simulink model "T37_v65_2015b"  (Simulink 8.6)
settings: Solver=ode45  StartTime=0.0  StopTime=180  FixedStep=0.001  MaxStep=0.1  RelTol=1e-3
values from neighbouring files (symbols this model uses):
  Aero_RP = Aero_RP*[-1 0 0;0 1 0;0 0 -1]    [t37_data.m]
  aileron_limits = [-0.35 0.35]*pi/180    [t37_data.m]
  CD_alpha = 0.3840    (= 0.384)    [t37_data.m]
  CD_beta = [-1.5700	1.2300 ... (first row only)    [t37_data.m]
  CD_flap = 0.0750    (= 0.075)    [t37_data.m]
  CD_zero = [  -1.5700	1.5000 ... (first row only)    [t37_data.m]
  Cl_ail = [0.0000	0.1810 ... (first row only)    [t37_data.m]
  CL_alpha = [-0.2000	-0.6400 ... (first row only)    [t37_data.m]
  CL_alpha_dot = 2.0    (= 2)    [t37_data.m]
  Cl_beta = -0.0944    [t37_data.m]
  CL_elev = 0.5    [t37_data.m]
  CL_flap = 0.3500    (= 0.35)    [t37_data.m]
  CL_ground_effect = [0.0000	1.0610 ... (first row only)    [t37_data.m]
  Cl_p = -0.4420    (= -0.442)    [t37_data.m]
  CL_q = 4.1    [t37_data.m]
  Cl_r = 0.0926    [t37_data.m]
  Cl_rudder = 0.0150    (= 0.015)    [t37_data.m]
  Cm_alpha = -0.7000    (= -0.7)    [t37_data.m]
  Cm_alpha_dot = -6.9500    (= -6.95)    [t37_data.m]
  Cm_elev = [0.0000	-1.1200 ... (first row only)    [t37_data.m]
  Cm_q = -50.0000    (= -50)    [t37_data.m]
  Cm_zero = 0.0250    (= 0.025)    [t37_data.m]
  Cn_beta = 0.1106    [t37_data.m]
  Cn_p = -0.0243    [t37_data.m]
  Cn_r = -0.1390    (= -0.139)    [t37_data.m]
  Cn_rudder = -0.0365    [t37_data.m]
  CY_beta = -0.3460    (= -0.346)    [t37_data.m]
  CY_p = -0.0827    [t37_data.m]
  CY_r = 0.3000    (= 0.3)    [t37_data.m]
  CY_rudder = 0.200    (= 0.2)    [t37_data.m]
  elevator_limits = [-0.35 0.3]*pi/180    [t37_data.m]
  isTrimming = 0    [mytrim.m]    (also in t37_data.m)
  Jxx = 7985*1.3558179    (= 10826.2059315)    [t37_data.m]
  Jxz = 0    [t37_data.m]
  Jyy = 6000*1.3558179    (= 8134.9074)    [t37_data.m]
  Jzz = 11183*1.3558179    (= 15162.1115757)    [t37_data.m]
  M = 4056*0.45359237    (= 1839.77065272)    [t37_data.m]
  Rcg = Rcg*[-1 0 0;0 1 0;0 0 -1]    [t37_data.m]
  Rengine1 = Rengine1*[-1 0 0;0 1 0;0 0 -1]    [t37_data.m]
  Rengine2 = Rengine2*[-1 0 0;0 1 0;0 0 -1]    [t37_data.m]
  rudder_limits = [-0.35 0.35]*pi/180    [t37_data.m]
  Sw = 182*0.09290304    (= 16.90835328)    [t37_data.m]
  thrust_limits = [0 1]    [t37_data.m]
  Tmax = M*10    (= 18397.7065272)    [t37_data.m]
  u0 = [ ... (first row only)    [mytrim.m]    (also in t37_data.m = zeros(4,1))
  x0 = [ ... (first row only)    [mytrim.m]    (also in t37_data.m = zeros(12,1))
undefined symbols (not defined in the file or in its folder): CD_elevator
undefined symbols (not defined in the file): Bw, Cw
(part 1 of 2)
settings Model: Creator=torres  LastModifiedBy=Pc melhor q do euler  ExtModeAutoUpdateStatusClock=off
settings DataIOCC: SaveOutput=off  SaveTime=off  SignalLoggingName=sigsOut
settings OptimizationCC: ExpressionDepthLimit=128  InitFltsAndDblsToZero=on
settings DebuggingCC: SaveWithParameterizedLinksMsg=none  SignalResolutionControl=TryResolveAllWithWarning  SolverPrmCheckMsg=none  MultiTaskDSMMsg=warning  MultiTaskCondExecSysMsg=none  FcnCallInpInsideContextMsg=EnableAllAsWarning  AllowSymbolicDim=on  StateNameClashWarn=none  StrictBusMsg=None
settings HardwareCC: TargetHWDeviceType=32-bit Generic  TargetUnknown=on  ProdEqTarget=off
settings GRTTargetCC: TargetFcnLib=ansi_tfl_tmw.mat  GeneratePreprocessorConditionals=Use local settings

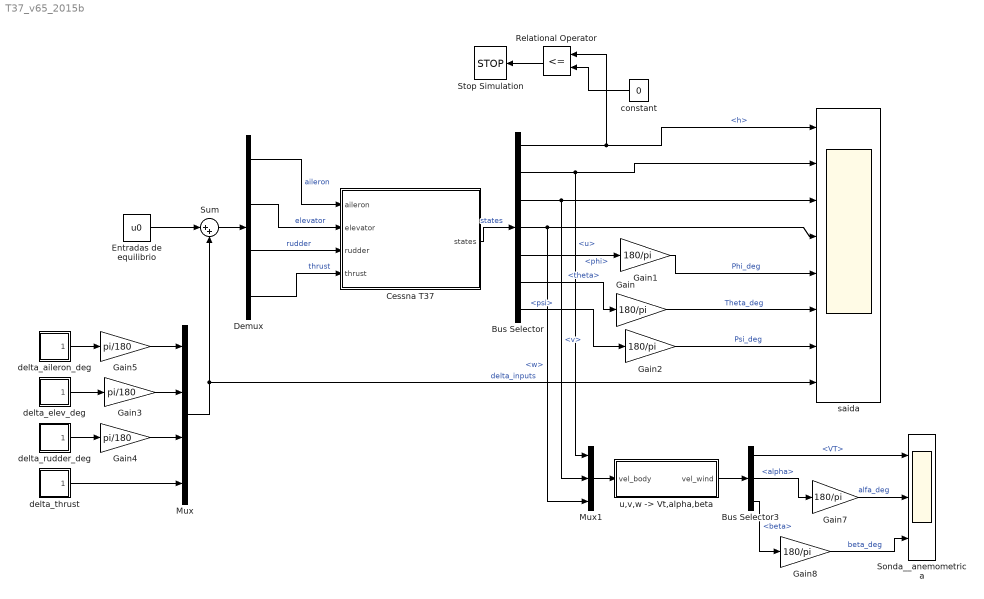
== system T37_v65_2015b ==
  Bus Selector : BusSelector  OutputSignals=h,u,v,w,phi,theta,psi
  Bus Selector3 : BusSelector  OutputSignals=VT,alpha,beta
  Cessna T37 : Subsystem
      mask Display: image(imread('c182.jpg'))
  Demux : Demux
  Entradas de equilibrio : Constant  Value=u0
  Gain{,1..2,7..8} (5 alike) : Gain  Gain=180/pi  SaturateOnIntegerOverflow=on  OutDataTypeStr=Inherit: Same as input  ParamDataTypeStr=Inherit: Same as input
  Gain3 : Gain  Gain=pi/180  SaturateOnIntegerOverflow=on  OutDataTypeStr=Inherit: Same as input  ParamDataTypeStr=Inherit: Same as input
  Gain4 : Gain  Gain=pi/180  SaturateOnIntegerOverflow=on  OutDataTypeStr=Inherit: Same as input  ParamDataTypeStr=Inherit: Same as input
  Gain5 : Gain  Gain=pi/180  SaturateOnIntegerOverflow=on  OutDataTypeStr=Inherit: Same as input  ParamDataTypeStr=Inherit: Same as input
  Mux : Mux
  Mux1 : Mux  Inputs=3
  Relational Operator : RelationalOperator  Operator=<=
  Sonda__anemometrica : Scope  NumInputPorts=3
  Stop Simulation : Stop
  Sum : Sum  Inputs=|++  SaturateOnIntegerOverflow=on
  constant : Constant  Value=0
  delta_aileron_deg : Subsystem  mask{t0=90, dt=5, A=1}
      mask prompts: t0 "Start time"; dt "Pulse Width"; A "Amplitude"
      mask help: Doublet input to control surface.
      mask Display: plot(0,0,100,100,[90,70,70,50,50,30,30,10],[50,50,10,10,90,90,50,50])
  delta_elev_deg : Subsystem  mask{t0=15, dt=1, A=-5}
      mask prompts: t0 "Start time"; dt "Pulse Width"; A "Amplitude"
      mask help: Doublet input to control surface.
      mask Display: plot(0,0,100,100,[90,70,70,50,50,30,30,10],[50,50,10,10,90,90,50,50])
  delta_rudder_deg : Subsystem  mask{t0=90, dt=1, A=0}
      mask prompts: t0 "Start time"; dt "Pulse Width"; A "Amplitude"
      mask help: Doublet input to control surface.
      mask Display: plot(0,0,100,100,[90,70,70,50,50,30,30,10],[50,50,10,10,90,90,50,50])
  delta_thrust : Subsystem  mask{t0=60, dt=1000, A=0}
      mask prompts: t0 "Start time"; dt "Duration"; A "Amplitude"
      mask Display: plot(0,0,100,100,[98,50,50,30,30,2],[20,20,80,80,20,20])
  saida : Scope  NumInputPorts=8
  "u,v,w -> Vt,alpha,beta" : Subsystem
  wires:
  Cessna T37/1(states) -> Bus Selector/1  "states"
  Bus Selector/2 -> saida/2, Mux1/1  "<u>"
  Bus Selector/3 -> saida/3, Mux1/2  "<v>"
  Bus Selector/4 -> saida/4, Mux1/3  "<w>"
  Bus Selector/5 -> Gain1/1  "<phi>"
  Bus Selector/6 -> Gain/1  "<theta>"
  Bus Selector/7 -> Gain2/1  "<psi>"
  Demux/1 -> Cessna T37/1(aileron)  "aileron"
  Gain/1 -> saida/6  "Theta_deg"
  Gain1/1 -> saida/5  "Phi_deg"
  Gain2/1 -> saida/7  "Psi_deg"
  Demux/2 -> Cessna T37/2(elevator)  "elevator"
  Demux/3 -> Cessna T37/3(rudder)  "rudder"
  Demux/4 -> Cessna T37/4(thrust)  "thrust"
  Entradas de equilibrio/1 -> Sum/1
  Sum/1 -> Demux/1
  delta_aileron_deg/1(Out1) -> Gain5/1
  delta_elev_deg/1(Out1) -> Gain3/1
  delta_rudder_deg/1(Out1) -> Gain4/1
  delta_thrust/1(Out1) -> Mux/4
  Mux/1 -> Sum/2, saida/8  "delta_inputs"
  Gain3/1 -> Mux/2
  Gain4/1 -> Mux/3
  Gain5/1 -> Mux/1
  Relational Operator/1 -> Stop Simulation/1
  constant/1 -> Relational Operator/2
  Bus Selector/1 -> saida/1, Relational Operator/1  "<h>"
  "u,v,w -> Vt,alpha,beta"/1(vel_wind) -> Bus Selector3/1
  Mux1/1 -> "u,v,w -> Vt,alpha,beta"/1(vel_body)
  Bus Selector3/1 -> Sonda__anemometrica/1  "<VT>"
  Bus Selector3/2 -> Gain7/1  "<alpha>"
  Bus Selector3/3 -> Gain8/1  "<beta>"
  Gain7/1 -> Sonda__anemometrica/2  "alfa_deg"
  Gain8/1 -> Sonda__anemometrica/3  "beta_deg"

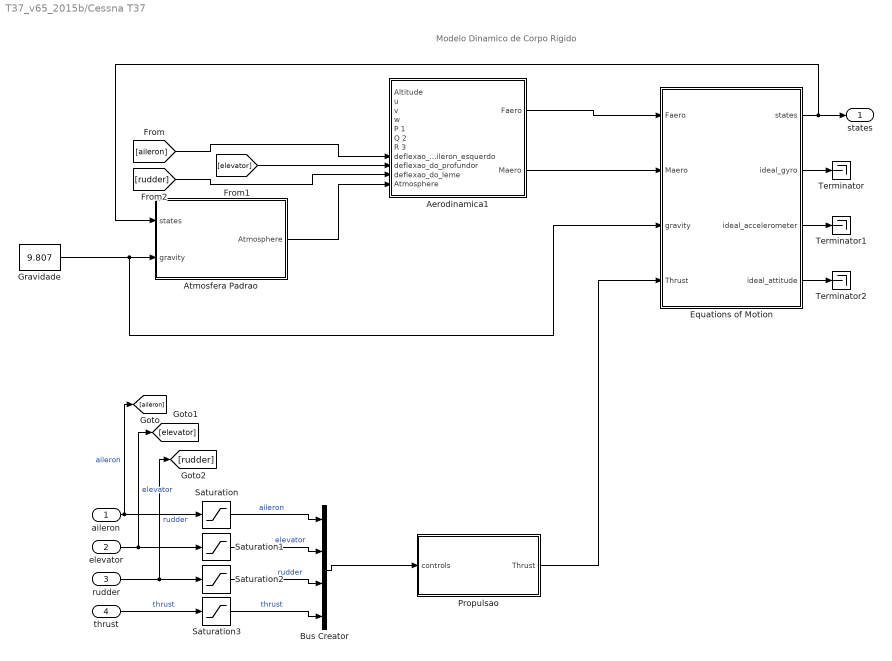
== system T37_v65_2015b/Cessna T37 ==
  note: Modelo Dinamico de Corpo Rigido
  aileron : Inport
  elevator : Inport  Port=2
  rudder : Inport  Port=3
  thrust : Inport  Port=4
  Aerodinamica1 : Subsystem  mask{flap=0, bw=Bw, cw=Cw, Sw=Sw}
      mask prompts: flap "Comando Flap (0, 1, 2 ou 3)"; bw "Comprimento da asa  - wingspan (m)"; cw "Corda media da asa (m)"; Sw "Area da asa (m2)"
  Atmosfera Padrao : Subsystem
  Bus Creator : BusCreator  Inputs=4
  Equations of Motion : Subsystem  mask{R_engine1=Rengine1, R_engine2=Rengine2, Rcg=Rcg, Aero_RP=Aero_RP, m=M, Jxz=Jxz, Jxx=Jxx, Jyy=Jyy, Jzz=Jzz, d=[0; 0; 0]}
      mask prompts: R_engine1 "Engine 1 position (row vector in meters)"; R_engine2 "Engine 2 position (row vector in meters)"; Rcg "C.G. position (m)"; Aero_RP "Nominal C.G. (m) = Aerodynamic Reference Point"; m "Aircraft mass (Kg)"; Jxz "Inertia product (Jxz)"; Jxx "Inertia (Jxx)"; Jyy "Inertia (Jyy)"; Jzz "Inertia (Jzz)"; d "Accelerometers displacement from CG (vector in the ABC frame, in (m))"
  Gravidade : Constant  Value=9.807
  Propulsao : Subsystem  mask{Tmax=Tmax}
      mask prompts: Tmax "Tracao Maxima (N)"
  Saturation : Saturate  UpperLimit=aileron_limits(2)  LowerLimit=aileron_limits(1)
  Saturation1 : Saturate  UpperLimit=elevator_limits(2)  LowerLimit=elevator_limits(1)
  Saturation2 : Saturate  UpperLimit=rudder_limits(2)  LowerLimit=rudder_limits(1)
  Saturation3 : Saturate  UpperLimit=thrust_limits(2)  LowerLimit=thrust_limits(1)
  Terminator : Terminator
  Terminator1 : Terminator
  Terminator2 : Terminator
  states : Outport
  wires:
  Equations of Motion/1(states) -> states/1, Atmosfera Padrao/1(states)
  aileron/1 -> [aileron], Saturation/1  "aileron"
  elevator/1 -> [elevator], Saturation1/1  "elevator"
  rudder/1 -> [rudder], Saturation2/1  "rudder"
  Gravidade/1 -> Atmosfera Padrao/2(gravity), Equations of Motion/3(gravity)
  thrust/1 -> Saturation3/1  "thrust"
  Bus Creator/1 -> Propulsao/1(controls)
  Propulsao/1(Thrust) -> Equations of Motion/4(Thrust)
  Saturation/1 -> Bus Creator/1  "aileron"
  Saturation1/1 -> Bus Creator/2  "elevator"
  Saturation2/1 -> Bus Creator/3  "rudder"
  Saturation3/1 -> Bus Creator/4  "thrust"
  Equations of Motion/2(ideal_gyro) -> Terminator/1
  Equations of Motion/4(ideal_attitude) -> Terminator2/1
  Equations of Motion/3(ideal_accelerometer) -> Terminator1/1
  Aerodinamica1/1(Faero) -> Equations of Motion/1(Faero)
  Aerodinamica1/2(Maero) -> Equations of Motion/2(Maero)
  Atmosfera Padrao/1(Atmosphere) -> Aerodinamica1/11(Atmosphere)
  [aileron] -> Aerodinamica1/8("deflexao_do_aileron_esquerdo ")
  [elevator] -> Aerodinamica1/9("deflexao_do_profundor ")
  [rudder] -> Aerodinamica1/10(deflexao_do_leme)

== system T37_v65_2015b/delta_aileron_deg ==
  Step : Step  Time=t0  After=A  SampleTime=0
  Step1 : Step  Time=t0+dt  After=-2*A  SampleTime=0
  Step2 : Step  Time=t0+2*dt  After=A  SampleTime=0
  Sum : Sum  Inputs=|++  SaturateOnIntegerOverflow=on
  Sum1 : Sum  Inputs=|++  SaturateOnIntegerOverflow=on
  Out1 : Outport
  wires:
  Step/1 -> Sum/1
  Step1/1 -> Sum/2
  Sum/1 -> Sum1/1
  Sum1/1 -> Out1/1
  Step2/1 -> Sum1/2

== system T37_v65_2015b/delta_elev_deg ==
  Step : Step  Time=t0  After=A  SampleTime=0
  Step1 : Step  Time=t0+dt  After=-2*A  SampleTime=0
  Step2 : Step  Time=t0+2*dt  After=A  SampleTime=0
  Sum : Sum  Inputs=|++  SaturateOnIntegerOverflow=on
  Sum1 : Sum  Inputs=|++  SaturateOnIntegerOverflow=on
  Out1 : Outport
  wires:
  Step/1 -> Sum/1
  Step1/1 -> Sum/2
  Sum/1 -> Sum1/1
  Sum1/1 -> Out1/1
  Step2/1 -> Sum1/2

== system T37_v65_2015b/delta_rudder_deg ==
  Step : Step  Time=t0  After=A  SampleTime=0
  Step1 : Step  Time=t0+dt  After=-2*A  SampleTime=0
  Step2 : Step  Time=t0+2*dt  After=A  SampleTime=0
  Sum : Sum  Inputs=|++  SaturateOnIntegerOverflow=on
  Sum1 : Sum  Inputs=|++  SaturateOnIntegerOverflow=on
  Out1 : Outport
  wires:
  Step/1 -> Sum/1
  Step1/1 -> Sum/2
  Sum/1 -> Sum1/1
  Sum1/1 -> Out1/1
  Step2/1 -> Sum1/2

== system T37_v65_2015b/delta_thrust ==
  Step : Step  Time=t0  After=A  SampleTime=0
  Step1 : Step  Time=t0+dt  After=-A  SampleTime=0
  Sum : Sum  Inputs=|++  SaturateOnIntegerOverflow=on
  Out1 : Outport
  wires:
  Sum/1 -> Out1/1
  Step/1 -> Sum/1
  Step1/1 -> Sum/2

== system T37_v65_2015b/u,v,w -> Vt,alpha,beta ==
  vel_body : Inport
  Bus Creator : BusCreator  Inputs=3
  VT : Fcn  Expr=sqrt(u(1)^2+u(2)^2+u(3)^2)
  alpha : Fcn  Expr=atan2(u(3),u(1))
  beta : Fcn  Expr=atan2(u(2),sqrt(u(1)^2+u(3)^2))
  vel_wind : Outport
  wires:
  Bus Creator/1 -> vel_wind/1
  VT/1 -> Bus Creator/1  "VT"
  alpha/1 -> Bus Creator/2  "alpha"
  vel_body/1 -> alpha/1, VT/1, beta/1
  beta/1 -> Bus Creator/3  "beta"

== system T37_v65_2015b/Cessna T37/Aerodinamica1 ==
  Altitude : Inport
  u : Inport  Port=2
  v : Inport  Port=3
  "w " : Inport  Port=4
  P 1 : Inport  Port=5
  Q 2 : Inport  Port=6
  R 3 : Inport  Port=7
  "deflexao_do_aileron_esquerdo " : Inport  Port=8
  "deflexao_do_profundor " : Inport  Port=9
  deflexao_do_leme : Inport  Port=10
  Atmosphere : Inport  Port=11
  Bus Selector1 : BusSelector  OutputSignals=densidade (Kg/m3)
  Bus Selector3 : BusSelector  OutputSignals=VT,alpha,beta
  Bus Selector4 : BusSelector  OutputSignals=VT,alpha,beta
  Forcas Aerodinamicas : Subsystem
  ForcasMomentos : Scope  NumInputPorts=2
  Momentos Aerodinamicos : Subsystem
  Mux : Mux  Inputs=3
  Wind->ABC : Subsystem
  "u,v,w -> Vt,alpha,beta" : Subsystem
  Faero : Outport
  Maero : Outport  Port=2
  wires:
  Bus Selector1/1 -> Momentos Aerodinamicos/10(densidade), Forcas Aerodinamicas/10(densidade)  "<densidade (Kg/m3)>"
  Altitude/1 -> Forcas Aerodinamicas/7(h)
  P 1/1 -> Forcas Aerodinamicas/4(p), Momentos Aerodinamicos/4(p)
  Q 2/1 -> Forcas Aerodinamicas/5(q), Momentos Aerodinamicos/5(q)
  R 3/1 -> Forcas Aerodinamicas/6(r), Momentos Aerodinamicos/6(r)
  "deflexao_do_aileron_esquerdo "/1 -> Momentos Aerodinamicos/9(aileron)
  "deflexao_do_profundor "/1 -> Momentos Aerodinamicos/8(elevator), Forcas Aerodinamicas/9(elevator)
  deflexao_do_leme/1 -> Momentos Aerodinamicos/7(rudder), Forcas Aerodinamicas/8(rudder)
  Bus Selector3/1 -> Forcas Aerodinamicas/1(VT)  "<VT>"
  Bus Selector3/2 -> Forcas Aerodinamicas/2(alpha), Wind->ABC/1(alpha)  "<alpha>"
  Bus Selector3/3 -> Forcas Aerodinamicas/3(beta), Wind->ABC/2(beta)  "<beta>"
  Bus Selector4/1 -> Momentos Aerodinamicos/1(VT)  "<VT>"
  Bus Selector4/2 -> Momentos Aerodinamicos/2(alpha)  "<alpha>"
  Bus Selector4/3 -> Momentos Aerodinamicos/3(beta)  "<beta>"
  "u,v,w -> Vt,alpha,beta"/1(vel_wind) -> Bus Selector3/1, Bus Selector4/1
  u/1 -> Mux/1
  v/1 -> Mux/2
  "w "/1 -> Mux/3
  Mux/1 -> "u,v,w -> Vt,alpha,beta"/1(vel_body)
  Forcas Aerodinamicas/1(Faero_wind) -> Wind->ABC/3(V_Wind), ForcasMomentos/1
  Wind->ABC/1(V_ABC) -> Faero/1
  Momentos Aerodinamicos/1(Maero_body) -> Maero/1, ForcasMomentos/2
  Atmosphere/1 -> Bus Selector1/1

== system T37_v65_2015b/Cessna T37/Atmosfera Padrao ==
  states : Inport
  gravity : Inport  Port=2
  Bus Creator : BusCreator  Inputs=4
  Bus Selector : BusSelector  OutputSignals=h
  Calc. Densidade : Fcn  Expr=1.225*(u(1)/288.15)^(-u(2)/(-0.0065*287.04)-1)
  Calc. Pressao : Fcn  Expr=101325*(u(1)/288.15)^(-u(2)/(-0.0065*287.04))
  Calc. Temperatura : Fcn  Expr=288.15 -0.0065*u(1)
  Calc. Vel. Som : Fcn  Expr=sqrt(u*1.4*287.04)
  Mux : Mux  Inputs=2
  Mux1 : Mux  Inputs=2
  Atmosphere : Outport
  wires:
  states/1 -> Bus Selector/1
  Bus Selector/1 -> Mux/1  "<h>"
  gravity/1 -> Mux/2, Mux1/2
  Mux/1 -> Calc. Temperatura/1
  Mux1/1 -> Calc. Pressao/1, Calc. Densidade/1
  Calc. Temperatura/1 -> Mux1/1, Calc. Vel. Som/1, Bus Creator/3  "Temperatura (K)"
  Calc. Pressao/1 -> Bus Creator/4  "Pressao (Pa)"
  Calc. Densidade/1 -> Bus Creator/1  "densidade (Kg/m3)"
  Calc. Vel. Som/1 -> Bus Creator/2  "Vel_som (m/s)"
  Bus Creator/1 -> Atmosphere/1

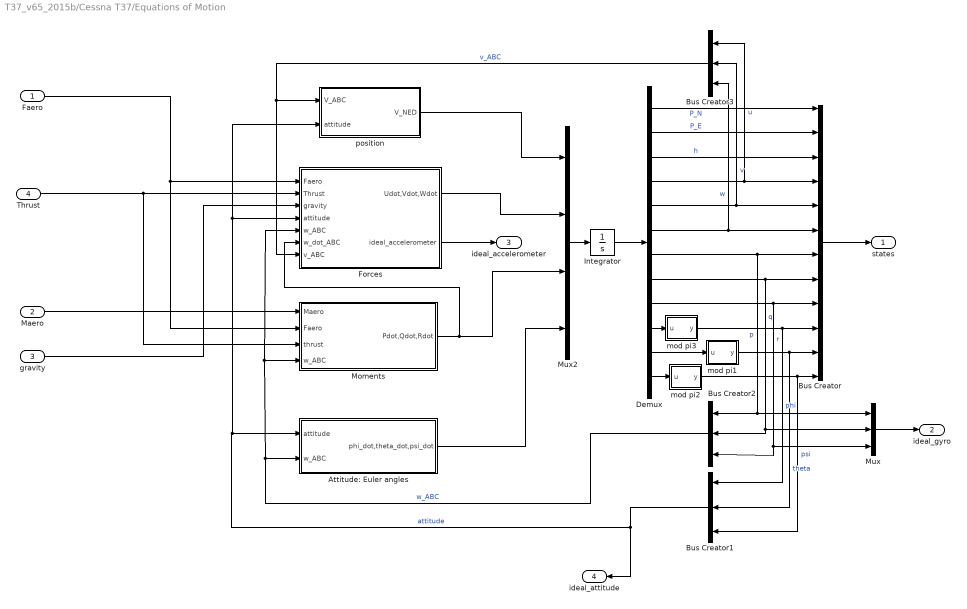
== system T37_v65_2015b/Cessna T37/Equations of Motion ==
  Faero : Inport
  Maero : Inport  Port=2
  gravity : Inport  Port=3
  Thrust : Inport  Port=4
  Attitude: Euler angles : Subsystem
  Bus Creator : BusCreator  Inputs=12
  Bus Creator1 : BusCreator  Inputs=3
  Bus Creator2 : BusCreator  Inputs=3
  Bus Creator3 : BusCreator  Inputs=3
  Demux : Demux  Outputs=12
  Forces : Subsystem
  Integrator : Integrator  InitialCondition=x0
  Moments : Subsystem
  Mux : Mux  Inputs=3
  Mux2 : Mux
  mod pi1 : Subsystem
  mod pi2 : Subsystem
  mod pi3 : Subsystem
  position : Subsystem
  states : Outport
  ideal_gyro : Outport  Port=2
  ideal_accelerometer : Outport  Port=3
  ideal_attitude : Outport  Port=4
  wires:
  Demux/3 -> Bus Creator/3  "h"
  Demux/4 -> Bus Creator/4, Bus Creator3/1  "u"
  Demux/5 -> Bus Creator/5, Bus Creator3/2  "v"
  Demux/6 -> Bus Creator/6, Bus Creator3/3  "w"
  Demux/7 -> Bus Creator/7, Bus Creator2/1, Mux/1  "p"
  Demux/8 -> Bus Creator/8, Bus Creator2/2, Mux/2  "q"
  Demux/9 -> Bus Creator/9, Bus Creator2/3, Mux/3  "r"
  Demux/10 -> mod pi3/1(u)
  Demux/11 -> mod pi1/1(u)
  Demux/12 -> mod pi2/1(u)
  Integrator/1 -> Demux/1
  Bus Creator/1 -> states/1
  Mux2/1 -> Integrator/1
  Thrust/1 -> Moments/3(thrust), Forces/2(Thrust)
  Bus Creator1/1 -> Attitude: Euler angles/1(attitude), Forces/4(attitude), position/2(attitude), ideal_attitude/1  "attitude"
  Forces/1(Udot,Vdot,Wdot) -> Mux2/2
  gravity/1 -> Forces/3(gravity)
  Attitude: Euler angles/1(phi_dot,theta_dot,psi_dot) -> Mux2/4
  Maero/1 -> Moments/1(Maero)
  Bus Creator3/1 -> Forces/7(v_ABC), position/1(V_ABC)  "v_ABC"
  Faero/1 -> Forces/1(Faero), Moments/2(Faero)
  Bus Creator2/1 -> Attitude: Euler angles/2(w_ABC), Forces/5(w_ABC), Moments/4(w_ABC)  "w_ABC"
  Moments/1(Pdot,Qdot,Rdot) -> Mux2/3, Forces/6(w_dot_ABC)
  Demux/1 -> Bus Creator/1  "P_N"
  Demux/2 -> Bus Creator/2  "P_E"
  position/1(V_NED) -> Mux2/1
  mod pi3/1(y) -> Bus Creator/10, Bus Creator1/1  "phi"
  mod pi1/1(y) -> Bus Creator/11, Bus Creator1/2  "theta"
  mod pi2/1(y) -> Bus Creator/12, Bus Creator1/3  "psi"
  Mux/1 -> ideal_gyro/1
  Forces/2(ideal_accelerometer) -> ideal_accelerometer/1

== system T37_v65_2015b/Cessna T37/Propulsao ==
  controls : Inport
  Bus Selector : BusSelector  OutputSignals=thrust
  Constant : Constant  Value=0
  Gain : Gain  Gain=Tmax  SaturateOnIntegerOverflow=on  OutDataTypeStr=Inherit: Same as input  ParamDataTypeStr=Inherit: Same as input
  Mux : Mux  Inputs=3
  Saturation : Saturate  UpperLimit=1  LowerLimit=0.0
  Thrust : Outport
  wires:
  Saturation/1 -> Gain/1
  controls/1 -> Bus Selector/1
  Bus Selector/1 -> Saturation/1  "<thrust>"
  Gain/1 -> Mux/1
  Mux/1 -> Thrust/1
  Constant/1 -> Mux/3, Mux/2

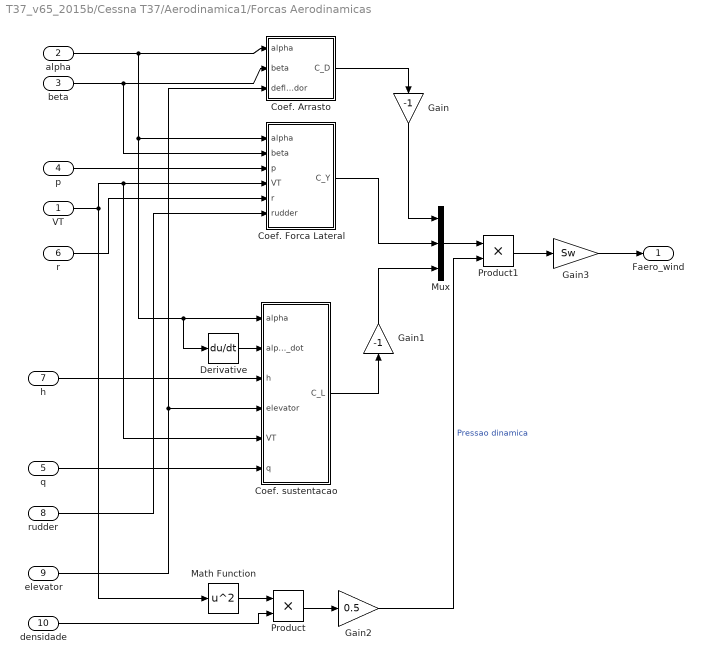
== system T37_v65_2015b/Cessna T37/Aerodinamica1/Forcas Aerodinamicas ==
  VT : Inport
  alpha : Inport  Port=2
  beta : Inport  Port=3
  p : Inport  Port=4
  q : Inport  Port=5
  r : Inport  Port=6
  h : Inport  Port=7
  rudder : Inport  Port=8
  elevator : Inport  Port=9
  densidade : Inport  Port=10
  Coef. Arrasto : Subsystem
  Coef. Forca Lateral : Subsystem
  Coef. sustentacao : Subsystem
  Derivative : Derivative
  Gain : Gain  Gain=-1  SaturateOnIntegerOverflow=on  OutDataTypeStr=Inherit: Same as input  ParamDataTypeStr=Inherit: Same as input
  Gain1 : Gain  Gain=-1  SaturateOnIntegerOverflow=on  OutDataTypeStr=Inherit: Same as input  ParamDataTypeStr=Inherit: Same as input
  Gain2 : Gain  Gain=0.5  SaturateOnIntegerOverflow=on  OutDataTypeStr=Inherit: Same as input  ParamDataTypeStr=Inherit: Same as input
  Gain3 : Gain  Gain=Sw  SaturateOnIntegerOverflow=on  OutDataTypeStr=Inherit: Same as input  ParamDataTypeStr=Inherit: Same as input
  Math Function : Math  Operator=square  SaturateOnIntegerOverflow=on
  Mux : Mux  Inputs=3
  Product : Product  SaturateOnIntegerOverflow=on  OutDataTypeStr=Inherit: Same as first input
  Product1 : Product  SaturateOnIntegerOverflow=on  OutDataTypeStr=Inherit: Same as first input
  Faero_wind : Outport
  wires:
  Coef. Arrasto/1(C_D) -> Gain/1
  Coef. Forca Lateral/1(C_Y) -> Mux/2
  alpha/1 -> Coef. Arrasto/1(alpha), Coef. Forca Lateral/1(alpha), Coef. sustentacao/1(alpha), Derivative/1
  beta/1 -> Coef. Arrasto/2(beta), Coef. Forca Lateral/2(beta)
  VT/1 -> Coef. Forca Lateral/4(VT), Coef. sustentacao/5(VT), Math Function/1
  p/1 -> Coef. Forca Lateral/3(p)
  q/1 -> Coef. sustentacao/6(q)
  r/1 -> Coef. Forca Lateral/5(r)
  h/1 -> Coef. sustentacao/3(h)
  rudder/1 -> Coef. Forca Lateral/6(rudder)
  elevator/1 -> Coef. Arrasto/3("deflexao_do_profundor "), Coef. sustentacao/4(elevator)
  Derivative/1 -> Coef. sustentacao/2(alpha_dot)
  Coef. sustentacao/1(C_L) -> Gain1/1
  Gain/1 -> Mux/1
  Gain1/1 -> Mux/3
  densidade/1 -> Product/2
  Math Function/1 -> Product/1
  Product/1 -> Gain2/1
  Mux/1 -> Product1/1
  Product1/1 -> Gain3/1
  Gain2/1 -> Product1/2  "Pressao dinamica"
  Gain3/1 -> Faero_wind/1

== system T37_v65_2015b/Cessna T37/Aerodinamica1/Momentos Aerodinamicos ==
  VT : Inport
  alpha : Inport  Port=2
  beta : Inport  Port=3
  p : Inport  Port=4
  q : Inport  Port=5
  r : Inport  Port=6
  rudder : Inport  Port=7
  elevator : Inport  Port=8
  aileron : Inport  Port=9
  densidade : Inport  Port=10
  Coef. arfagem x cw : Subsystem
  Coef. guinada x bw : Subsystem
  Coef. rolamento x bw : Subsystem
  Derivative : Derivative
  Gain2 : Gain  Gain=1/2  SaturateOnIntegerOverflow=on  OutDataTypeStr=Inherit: Same as input  ParamDataTypeStr=Inherit: Same as input
  Gain3 : Gain  Gain=Sw  SaturateOnIntegerOverflow=on  OutDataTypeStr=Inherit: Same as input  ParamDataTypeStr=Inherit: Same as input
  Math Function : Math  Operator=square  SaturateOnIntegerOverflow=on
  Mux : Mux  Inputs=3
  Pdyn : Scope
  Product : Product  SaturateOnIntegerOverflow=on  OutDataTypeStr=Inherit: Same as first input
  Product1 : Product  SaturateOnIntegerOverflow=on  OutDataTypeStr=Inherit: Same as first input
  Maero_body : Outport
  wires:
  alpha/1 -> Coef. rolamento x bw/1(alpha), Coef. arfagem x cw/1(alpha), Derivative/1, Coef. guinada x bw/1(alpha)
  beta/1 -> Coef. rolamento x bw/2(beta), Coef. guinada x bw/2(beta)
  VT/1 -> Coef. rolamento x bw/3(VT), Coef. arfagem x cw/3(VT), Coef. guinada x bw/4(VT), Math Function/1
  p/1 -> Coef. rolamento x bw/4(p), Coef. guinada x bw/3(p)
  r/1 -> Coef. rolamento x bw/5(r), Coef. guinada x bw/5(r)
  Derivative/1 -> Coef. arfagem x cw/2(alpha_dot)
  q/1 -> Coef. arfagem x cw/4(q)
  rudder/1 -> Coef. rolamento x bw/7(rudder), Coef. guinada x bw/6(rudder)
  elevator/1 -> Coef. arfagem x cw/5(elevator)
  aileron/1 -> Coef. rolamento x bw/6(aileron)
  Mux/1 -> Product1/1
  Product1/1 -> Gain3/1
  Coef. rolamento x bw/1(Cl_bw) -> Mux/1
  Coef. arfagem x cw/1(Cm_cw) -> Mux/2
  Coef. guinada x bw/1(Cn_bw) -> Mux/3
  densidade/1 -> Product/2
  Math Function/1 -> Product/1
  Product/1 -> Gain2/1
  Gain2/1 -> Product1/2, Pdyn/1  "Pressao dinamica"
  Gain3/1 -> Maero_body/1

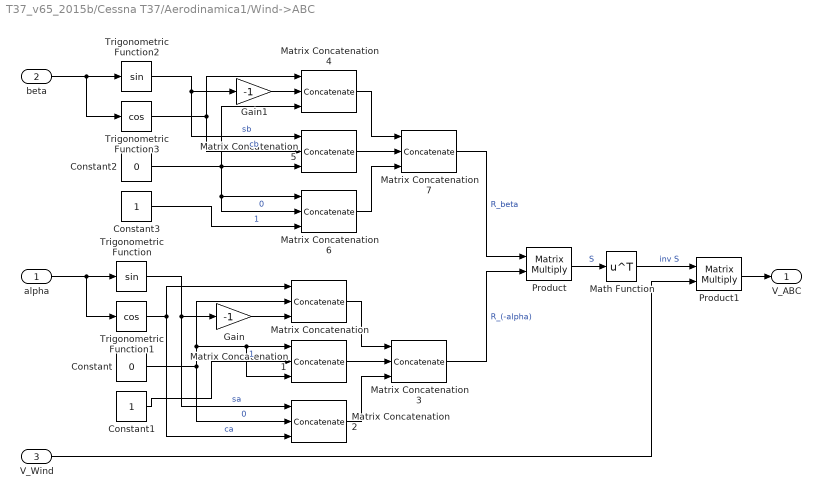
== system T37_v65_2015b/Cessna T37/Aerodinamica1/Wind->ABC ==
  alpha : Inport
  beta : Inport  Port=2
  V_Wind : Inport  Port=3
  Constant : Constant  Value=0
  Constant1 : Constant
  Constant2 : Constant  Value=0
  Constant3 : Constant
  Gain : Gain  Gain=-1  SaturateOnIntegerOverflow=on  OutDataTypeStr=Inherit: Same as input  ParamDataTypeStr=Inherit: Same as input
  Gain1 : Gain  Gain=-1  SaturateOnIntegerOverflow=on  OutDataTypeStr=Inherit: Same as input  ParamDataTypeStr=Inherit: Same as input
  Math Function : Math  Operator=transpose  SaturateOnIntegerOverflow=on
  Matrix Concatenation{,1..2,4..6} (6 alike) : Concatenate  NumInputs=3  Mode=Multidimensional array
  Matrix Concatenation3 : Concatenate  NumInputs=3  Mode=Multidimensional array  ConcatenateDimension=2
  Matrix Concatenation7 : Concatenate  NumInputs=3  Mode=Multidimensional array  ConcatenateDimension=2
  Product : Product  Multiplication=Matrix(*)  SaturateOnIntegerOverflow=on  OutDataTypeStr=Inherit: Same as first input
  Product1 : Product  Multiplication=Matrix(*)  SaturateOnIntegerOverflow=on  OutDataTypeStr=Inherit: Same as first input
  Trigonometric Function : Trigonometry
  Trigonometric Function1 : Trigonometry  Operator=cos
  Trigonometric Function2 : Trigonometry
  Trigonometric Function3 : Trigonometry  Operator=cos
  V_ABC : Outport
  wires:
  alpha/1 -> Trigonometric Function/1, Trigonometric Function1/1
  Trigonometric Function1/1 -> Matrix Concatenation/1, Matrix Concatenation2/3  "ca"
  Trigonometric Function/1 -> Matrix Concatenation2/1, Gain/1  "sa"
  Constant/1 -> Matrix Concatenation/2, Matrix Concatenation1/1, Matrix Concatenation1/3, Matrix Concatenation2/2  "0"
  Constant1/1 -> Matrix Concatenation1/2  "1"
  Matrix Concatenation/1 -> Matrix Concatenation3/1
  Matrix Concatenation1/1 -> Matrix Concatenation3/2
  Matrix Concatenation2/1 -> Matrix Concatenation3/3
  Product/1 -> Math Function/1  "S"
  Math Function/1 -> Product1/1  "inv S"
  Product1/1 -> V_ABC/1
  beta/1 -> Trigonometric Function2/1, Trigonometric Function3/1
  Matrix Concatenation4/1 -> Matrix Concatenation7/1
  Matrix Concatenation5/1 -> Matrix Concatenation7/2
  Matrix Concatenation6/1 -> Matrix Concatenation7/3
  Trigonometric Function3/1 -> Matrix Concatenation4/1, Matrix Concatenation5/2  "cb"
  Trigonometric Function2/1 -> Gain1/1, Matrix Concatenation5/1  "sb"
  Constant2/1 -> Matrix Concatenation4/3, Matrix Concatenation5/3, Matrix Concatenation6/1, Matrix Concatenation6/2  "0"
  Constant3/1 -> Matrix Concatenation6/3  "1"
  Matrix Concatenation7/1 -> Product/1  "R_beta"
  Matrix Concatenation3/1 -> Product/2  "R_(-alpha)"
  Gain1/1 -> Matrix Concatenation4/2
  V_Wind/1 -> Product1/2
  Gain/1 -> Matrix Concatenation/3

== system T37_v65_2015b/Cessna T37/Aerodinamica1/u,v,w -> Vt,alpha,beta ==
  vel_body : Inport
  Bus Creator : BusCreator  Inputs=3
  VT : Fcn  Expr=sqrt(u(1)^2+u(2)^2+u(3)^2)
  alpha : Fcn  Expr=atan2(u(3),u(1))
  beta : Fcn  Expr=atan2(u(2),sqrt(u(1)^2+u(3)^2))
  vel_wind : Outport
  wires:
  Bus Creator/1 -> vel_wind/1
  VT/1 -> Bus Creator/1  "VT"
  alpha/1 -> Bus Creator/2  "alpha"
  vel_body/1 -> alpha/1, VT/1, beta/1
  beta/1 -> Bus Creator/3  "beta"

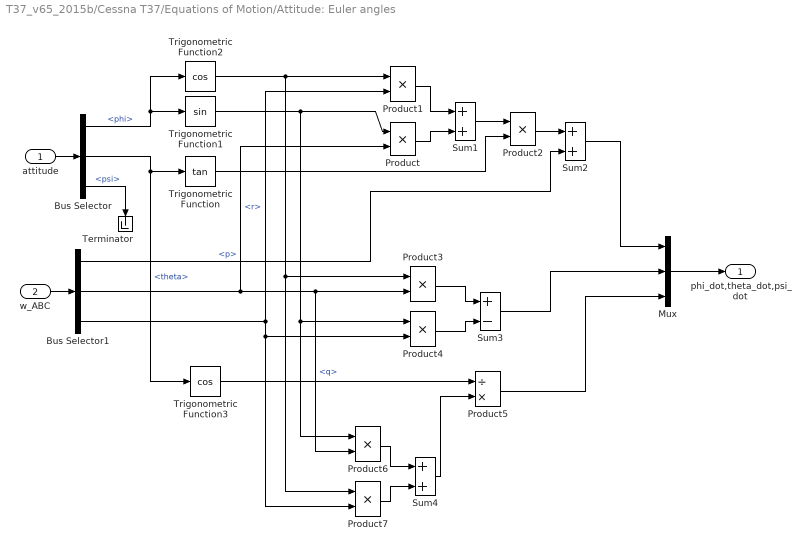
== system T37_v65_2015b/Cessna T37/Equations of Motion/Attitude: Euler angles ==
  attitude : Inport
  w_ABC : Inport  Port=2
  Bus Selector : BusSelector  OutputSignals=phi,theta,psi
  Bus Selector1 : BusSelector  OutputSignals=p,q,r
  Mux : Mux  Inputs=3
  Product{,1..4,6..7} (7 alike) : Product  SaturateOnIntegerOverflow=on  OutDataTypeStr=Inherit: Same as first input
  Product5 : Product  Inputs=/*  SaturateOnIntegerOverflow=on  OutDataTypeStr=Inherit: Same as first input
  Sum1 : Sum  SaturateOnIntegerOverflow=on
  Sum2 : Sum  SaturateOnIntegerOverflow=on
  Sum3 : Sum  Inputs=+-  SaturateOnIntegerOverflow=on
  Sum4 : Sum  SaturateOnIntegerOverflow=on
  Terminator : Terminator
  Trigonometric Function : Trigonometry  Operator=tan
  Trigonometric Function1 : Trigonometry
  Trigonometric Function2 : Trigonometry  Operator=cos
  Trigonometric Function3 : Trigonometry  Operator=cos
  phi_dot,theta_dot,psi_dot : Outport
  wires:
  Bus Selector/2 -> Trigonometric Function3/1, Trigonometric Function/1  "<theta>"
  Bus Selector/1 -> Trigonometric Function1/1, Trigonometric Function2/1  "<phi>"
  Trigonometric Function1/1 -> Product/1, Product4/1, Product6/1
  Trigonometric Function2/1 -> Product1/1, Product3/1, Product7/1
  Product1/1 -> Sum1/1
  Product/1 -> Sum1/2
  Sum1/1 -> Product2/1
  Product2/1 -> Sum2/1
  Sum2/1 -> Mux/1
  attitude/1 -> Bus Selector/1
  Bus Selector/3 -> Terminator/1  "<psi>"
  Product3/1 -> Sum3/1
  w_ABC/1 -> Bus Selector1/1
  Product4/1 -> Sum3/2
  Trigonometric Function3/1 -> Product5/1
  Product6/1 -> Sum4/1
  Product7/1 -> Sum4/2
  Sum4/1 -> Product5/2
  Sum3/1 -> Mux/2
  Product5/1 -> Mux/3
  Bus Selector1/1 -> Sum2/2  "<p>"
  Mux/1 -> phi_dot,theta_dot,psi_dot/1
  Bus Selector1/2 -> Product/2, Product3/2, Product6/2  "<q>"
  Bus Selector1/3 -> Product1/2, Product4/2, Product7/2  "<r>"
  Trigonometric Function/1 -> Product2/2

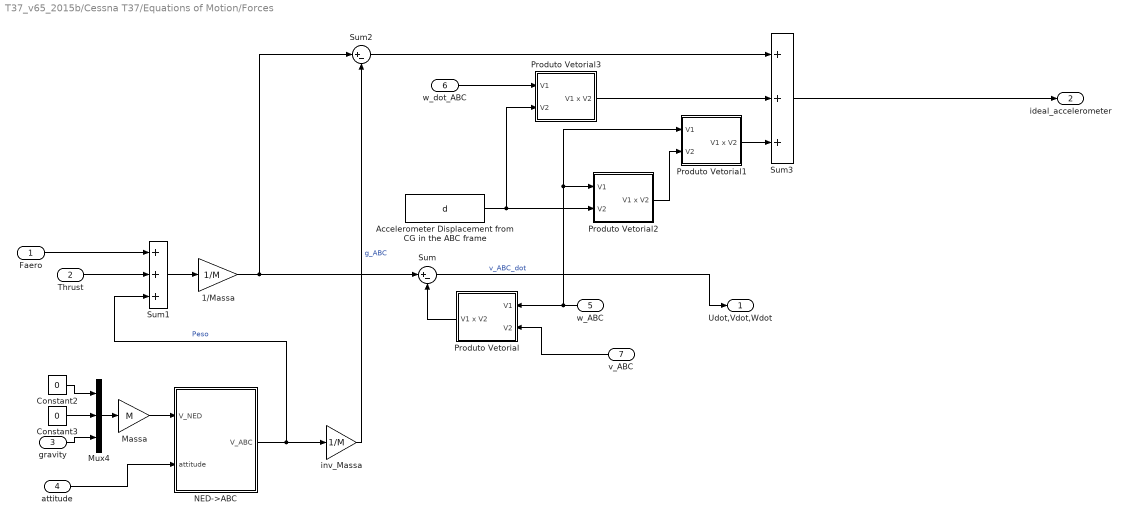
== system T37_v65_2015b/Cessna T37/Equations of Motion/Forces ==
  Faero : Inport
  Thrust : Inport  Port=2
  gravity : Inport  Port=3
  attitude : Inport  Port=4
  w_ABC : Inport  Port=5
  w_dot_ABC : Inport  Port=6
  v_ABC : Inport  Port=7
  1/Massa : Gain  Gain=1/M  SaturateOnIntegerOverflow=on  OutDataTypeStr=Inherit: Same as input  ParamDataTypeStr=Inherit: Same as input
  Accelerometer Displacement from CG in the ABC frame : Constant  Value=d
  Constant2 : Constant  Value=0
  Constant3 : Constant  Value=0
  Massa : Gain  Gain=M  SaturateOnIntegerOverflow=on  OutDataTypeStr=Inherit: Same as input  ParamDataTypeStr=Inherit: Same as input
  Mux4 : Mux  Inputs=3
  NED->ABC : Subsystem
  Produto Vetorial : Subsystem
  Produto Vetorial1 : Subsystem
  Produto Vetorial2 : Subsystem
  Produto Vetorial3 : Subsystem
  Sum : Sum  Inputs=|+-  SaturateOnIntegerOverflow=on
  Sum1 : Sum  Inputs=+++  SaturateOnIntegerOverflow=on
  Sum2 : Sum  Inputs=|+-  SaturateOnIntegerOverflow=on
  Sum3 : Sum  Inputs=+++  SaturateOnIntegerOverflow=on
  inv_Massa : Gain  Gain=1/M  SaturateOnIntegerOverflow=on  OutDataTypeStr=Inherit: Same as input  ParamDataTypeStr=Inherit: Same as input
  Udot,Vdot,Wdot : Outport
  ideal_accelerometer : Outport  Port=2
  wires:
  1/Massa/1 -> Sum/1, Sum2/1
  Produto Vetorial/1(V1 x V2) -> Sum/2
  w_ABC/1 -> Produto Vetorial/1(V1), Produto Vetorial2/1(V1), Produto Vetorial1/1(V1)
  v_ABC/1 -> Produto Vetorial/2(V2)
  Sum1/1 -> 1/Massa/1
  Constant2/1 -> Mux4/1
  Constant3/1 -> Mux4/2
  gravity/1 -> Mux4/3
  Mux4/1 -> Massa/1
  Massa/1 -> NED->ABC/1(V_NED)
  attitude/1 -> NED->ABC/2(attitude)
  Faero/1 -> Sum1/1
  Thrust/1 -> Sum1/2
  Sum/1 -> Udot,Vdot,Wdot/1  "v_ABC_dot"
  NED->ABC/1(V_ABC) -> Sum1/3, inv_Massa/1  "Peso"
  inv_Massa/1 -> Sum2/2  "g_ABC"
  Sum2/1 -> Sum3/1
  Sum3/1 -> ideal_accelerometer/1
  Produto Vetorial2/1(V1 x V2) -> Produto Vetorial1/2(V2)
  Accelerometer Displacement from CG in the ABC frame/1 -> Produto Vetorial2/2(V2), Produto Vetorial3/2(V2)
  Produto Vetorial1/1(V1 x V2) -> Sum3/3
  Produto Vetorial3/1(V1 x V2) -> Sum3/2
  w_dot_ABC/1 -> Produto Vetorial3/1(V1)

== system T37_v65_2015b/Cessna T37/Equations of Motion/Moments ==
  Maero : Inport
  Faero : Inport  Port=2
  thrust : Inport  Port=3
  w_ABC : Inport  Port=4
  Aerodynamic Forces  point of application : Constant  Value=Aero_RP
  C.G. position : Constant  Value=Rcg
  Engine position : Constant  Value=Rengine1
  Engine position 2 : Constant  Value=Rengine2
  Inertia : Subsystem
  Inverse Inertia Matrix : Subsystem
  Product : Product  Multiplication=Matrix(*)  SaturateOnIntegerOverflow=on  OutDataTypeStr=Inherit: Same as first input
  Product1 : Product  Multiplication=Matrix(*)  SaturateOnIntegerOverflow=on  OutDataTypeStr=Inherit: Same as first input
  Product2 : Product  Multiplication=Matrix(*)  SaturateOnIntegerOverflow=on  OutDataTypeStr=Inherit: Same as first input
  Produto Vetorial1 : Subsystem
  Produto Vetorial2 : Subsystem
  Produto Vetorial3 : Subsystem
  Produto Vetorial4 : Subsystem
  Sum1 : Sum  Inputs=|+-  SaturateOnIntegerOverflow=on
  Sum2 : Sum  Inputs=++++  SaturateOnIntegerOverflow=on
  Sum3 : Sum  Inputs=|+-  SaturateOnIntegerOverflow=on
  Sum4 : Sum  Inputs=|-+  SaturateOnIntegerOverflow=on
  Sum5 : Sum  Inputs=|+-  SaturateOnIntegerOverflow=on
  Pdot,Qdot,Rdot : Outport
  wires:
  Inverse Inertia Matrix/1(inv J) -> Product/1, Product2/1
  Sum2/1 -> Product/2
  Product/1 -> Sum3/1
  Inertia/1(J) -> Product1/1
  w_ABC/1 -> Product1/2, Produto Vetorial1/1(V1)
  Product1/1 -> Produto Vetorial1/2(V2)
  Produto Vetorial1/1(V1 x V2) -> Product2/2
  Product2/1 -> Sum3/2
  C.G. position/1 -> Sum5/2, Sum1/2, Sum4/1
  Aerodynamic Forces  point of application/1 -> Sum4/2
  Sum5/1 -> Produto Vetorial2/1(V1)
  Sum4/1 -> Produto Vetorial3/1(V1)
  Faero/1 -> Produto Vetorial3/2(V2)
  Produto Vetorial3/1(V1 x V2) -> Sum2/3
  Produto Vetorial2/1(V1 x V2) -> Sum2/2
  thrust/1 -> Produto Vetorial4/2(V2), Produto Vetorial2/2(V2)
  Sum3/1 -> Pdot,Qdot,Rdot/1
  Maero/1 -> Sum2/1
  Engine position/1 -> Sum5/1
  Produto Vetorial4/1(V1 x V2) -> Sum2/4
  Engine position 2/1 -> Sum1/1
  Sum1/1 -> Produto Vetorial4/1(V1)

== system T37_v65_2015b/Cessna T37/Equations of Motion/mod pi1 ==
  u : Inport
  Abs : Abs  SaturateOnIntegerOverflow=on
  Constant : Constant  Value=pi
  Fcn : Fcn  Expr=u/pi
  Fcn1 : Fcn  Expr=u*pi
  Gain : Gain  Gain=1/2  SaturateOnIntegerOverflow=on  OutDataTypeStr=Inherit: Same as input  ParamDataTypeStr=Inherit: Same as input
  Gain1 : Gain  Gain=2  SaturateOnIntegerOverflow=on  OutDataTypeStr=Inherit: Same as input  ParamDataTypeStr=Inherit: Same as input
  Product : Product  SaturateOnIntegerOverflow=on  OutDataTypeStr=Inherit: Same as first input
  Rounding Function : Rounding  Operator=fix
  Rounding Function1 : Rounding  Operator=fix
  Sign : Signum
  Sum : Sum  Inputs=|-+  SaturateOnIntegerOverflow=on
  Sum1 : Sum  Inputs=-+|  SaturateOnIntegerOverflow=on
  Sum2 : Sum  Inputs=+-|  SaturateOnIntegerOverflow=on
  Switch1 : Switch  Threshold=0.5  SaturateOnIntegerOverflow=on
  y : Outport
  wires:
  u/1 -> Abs/1, Sign/1
  Fcn/1 -> Rounding Function/1
  Rounding Function/1 -> Fcn1/1, Gain/1, Sum2/1
  Fcn1/1 -> Sum/1
  Abs/1 -> Fcn/1, Sum/2
  Sign/1 -> Product/2
  Product/1 -> y/1
  Sum/1 -> Sum1/2, Switch1/3
  Constant/1 -> Sum1/1
  Sum1/1 -> Switch1/1
  Switch1/1 -> Product/1
  Gain/1 -> Rounding Function1/1
  Rounding Function1/1 -> Gain1/1
  Gain1/1 -> Sum2/2
  Sum2/1 -> Switch1/2

== system T37_v65_2015b/Cessna T37/Equations of Motion/mod pi2 ==
  u : Inport
  Abs : Abs  SaturateOnIntegerOverflow=on
  Constant : Constant  Value=pi
  Fcn : Fcn  Expr=u/pi
  Fcn1 : Fcn  Expr=u*pi
  Gain : Gain  Gain=1/2  SaturateOnIntegerOverflow=on  OutDataTypeStr=Inherit: Same as input  ParamDataTypeStr=Inherit: Same as input
  Gain1 : Gain  Gain=2  SaturateOnIntegerOverflow=on  OutDataTypeStr=Inherit: Same as input  ParamDataTypeStr=Inherit: Same as input
  Product : Product  SaturateOnIntegerOverflow=on  OutDataTypeStr=Inherit: Same as first input
  Rounding Function : Rounding  Operator=fix
  Rounding Function1 : Rounding  Operator=fix
  Sign : Signum
  Sum : Sum  Inputs=|-+  SaturateOnIntegerOverflow=on
  Sum1 : Sum  Inputs=-+|  SaturateOnIntegerOverflow=on
  Sum2 : Sum  Inputs=+-|  SaturateOnIntegerOverflow=on
  Switch1 : Switch  Threshold=0.5  SaturateOnIntegerOverflow=on
  y : Outport
  wires:
  u/1 -> Abs/1, Sign/1
  Fcn/1 -> Rounding Function/1
  Rounding Function/1 -> Fcn1/1, Gain/1, Sum2/1
  Fcn1/1 -> Sum/1
  Abs/1 -> Fcn/1, Sum/2
  Sign/1 -> Product/2
  Product/1 -> y/1
  Sum/1 -> Sum1/2, Switch1/3
  Constant/1 -> Sum1/1
  Sum1/1 -> Switch1/1
  Switch1/1 -> Product/1
  Gain/1 -> Rounding Function1/1
  Rounding Function1/1 -> Gain1/1
  Gain1/1 -> Sum2/2
  Sum2/1 -> Switch1/2

== system T37_v65_2015b/Cessna T37/Equations of Motion/mod pi3 ==
  u : Inport
  Abs : Abs  SaturateOnIntegerOverflow=on
  Constant : Constant  Value=pi
  Fcn : Fcn  Expr=u/pi
  Fcn1 : Fcn  Expr=u*pi
  Gain : Gain  Gain=1/2  SaturateOnIntegerOverflow=on  OutDataTypeStr=Inherit: Same as input  ParamDataTypeStr=Inherit: Same as input
  Gain1 : Gain  Gain=2  SaturateOnIntegerOverflow=on  OutDataTypeStr=Inherit: Same as input  ParamDataTypeStr=Inherit: Same as input
  Product : Product  SaturateOnIntegerOverflow=on  OutDataTypeStr=Inherit: Same as first input
  Rounding Function : Rounding  Operator=fix
  Rounding Function1 : Rounding  Operator=fix
  Sign : Signum
  Sum : Sum  Inputs=|-+  SaturateOnIntegerOverflow=on
  Sum1 : Sum  Inputs=-+|  SaturateOnIntegerOverflow=on
  Sum2 : Sum  Inputs=+-|  SaturateOnIntegerOverflow=on
  Switch1 : Switch  Threshold=0.5  SaturateOnIntegerOverflow=on
  y : Outport
  wires:
  u/1 -> Abs/1, Sign/1
  Fcn/1 -> Rounding Function/1
  Rounding Function/1 -> Fcn1/1, Gain/1, Sum2/1
  Fcn1/1 -> Sum/1
  Abs/1 -> Fcn/1, Sum/2
  Sign/1 -> Product/2
  Product/1 -> y/1
  Sum/1 -> Sum1/2, Switch1/3
  Constant/1 -> Sum1/1
  Sum1/1 -> Switch1/1
  Switch1/1 -> Product/1
  Gain/1 -> Rounding Function1/1
  Rounding Function1/1 -> Gain1/1
  Gain1/1 -> Sum2/2
  Sum2/1 -> Switch1/2

== system T37_v65_2015b/Cessna T37/Equations of Motion/position ==
  V_ABC : Inport
  attitude : Inport  Port=2
  ABC->NED : Subsystem
  Constant : Constant  Value=0  VectorParams1D=off
  Constant1 : Constant  Value=isTrimming  VectorParams1D=off
  Demux1 : Demux  Outputs=3
  Gain : Gain  Gain=-1  SaturateOnIntegerOverflow=on  OutDataTypeStr=Inherit: Same as input  ParamDataTypeStr=Inherit: Same as input
  Mux : Mux  Inputs=3
  Switch : Switch  Threshold=0.5  SaturateOnIntegerOverflow=on
  Switch1 : Switch  Threshold=0.5  SaturateOnIntegerOverflow=on
  V_NED : Outport
  wires:
  ABC->NED/1(V_NED) -> Demux1/1
  V_ABC/1 -> ABC->NED/1(V_ABC)
  attitude/1 -> ABC->NED/2(attitude)
  Demux1/3 -> Gain/1  "-h"
  Gain/1 -> Mux/3
  Mux/1 -> V_NED/1
  Switch/1 -> Mux/1
  Demux1/1 -> Switch/3  "V_N"
  Switch1/1 -> Mux/2
  Demux1/2 -> Switch1/3  "V_E"
  Constant/1 -> Switch/1, Switch1/1
  Constant1/1 -> Switch/2, Switch1/2

== system T37_v65_2015b/Cessna T37/Aerodinamica1/Forcas Aerodinamicas/Coef. Arrasto ==
  alpha : Inport
  beta : Inport  Port=2
  "deflexao_do_profundor " : Inport  Port=3
  CD_beta : Lookup  InputValues=CD_beta(:,1);  Table=CD_beta(:,2);  SaturateOnIntegerOverflow=on
  CD_zero : Lookup  InputValues=CD_zero(:,1);  Table=CD_zero(:,2);  SaturateOnIntegerOverflow=on
  Constant2 : Constant  Value=CD_flap
  Gain1 : Gain  Gain=CD_alpha  SaturateOnIntegerOverflow=on  OutDataTypeStr=Inherit: Same as input  ParamDataTypeStr=Inherit: Same as input
  Gain2 : Gain  Gain=CD_elevator  SaturateOnIntegerOverflow=on  OutDataTypeStr=Inherit: Same as input  ParamDataTypeStr=Inherit: Same as input
  Sum : Sum  Inputs=+++++  SaturateOnIntegerOverflow=on
  C_D : Outport
  wires:
  alpha/1 -> CD_zero/1, Gain1/1
  Constant2/1 -> Sum/4
  Sum/1 -> C_D/1
  CD_zero/1 -> Sum/1
  Gain1/1 -> Sum/2
  CD_beta/1 -> Sum/3
  beta/1 -> CD_beta/1
  Gain2/1 -> Sum/5
  "deflexao_do_profundor "/1 -> Gain2/1

== system T37_v65_2015b/Cessna T37/Aerodinamica1/Forcas Aerodinamicas/Coef. Forca Lateral ==
  alpha : Inport
  beta : Inport  Port=2
  p : Inport  Port=3
  VT : Inport  Port=4
  r : Inport  Port=5
  rudder : Inport  Port=6
  Constant2 : Constant  Value=bw
  Gain : Gain  Gain=CY_rudder  SaturateOnIntegerOverflow=on  OutDataTypeStr=Inherit: Same as input  ParamDataTypeStr=Inherit: Same as input
  Gain1 : Gain  Gain=2  SaturateOnIntegerOverflow=on  OutDataTypeStr=Inherit: Same as input  ParamDataTypeStr=Inherit: Same as input
  Gain2 : Gain  Gain=CY_beta  SaturateOnIntegerOverflow=on  OutDataTypeStr=Inherit: Same as input  ParamDataTypeStr=Inherit: Same as input
  Gain3 : Gain  Gain=CY_p  SaturateOnIntegerOverflow=on  OutDataTypeStr=Inherit: Same as input  ParamDataTypeStr=Inherit: Same as input
  Gain4 : Gain  Gain=CY_r  SaturateOnIntegerOverflow=on  OutDataTypeStr=Inherit: Same as input  ParamDataTypeStr=Inherit: Same as input
  Product : Product  SaturateOnIntegerOverflow=on  OutDataTypeStr=Inherit: Same as first input
  Product1 : Product  Inputs=3  SaturateOnIntegerOverflow=on  OutDataTypeStr=Inherit: Same as first input
  Product2 : Product  Inputs=3  SaturateOnIntegerOverflow=on  OutDataTypeStr=Inherit: Same as first input
  Product3 : Product  Inputs=*/  SaturateOnIntegerOverflow=on  OutDataTypeStr=Inherit: Same as first input
  Sum : Sum  Inputs=++++  SaturateOnIntegerOverflow=on
  C_Y : Outport
  wires:
  alpha/1 -> Gain2/1, Gain4/1, Gain3/1
  beta/1 -> Product/2
  Sum/1 -> C_Y/1
  Product/1 -> Sum/1
  Product1/1 -> Sum/2
  Gain3/1 -> Product1/1
  p/1 -> Product1/2
  VT/1 -> Gain1/1
  Gain1/1 -> Product3/2
  Constant2/1 -> Product3/1
  Product3/1 -> Product1/3, Product2/1
  Product2/1 -> Sum/3
  r/1 -> Product2/3
  Gain/1 -> Sum/4
  rudder/1 -> Gain/1
  Gain2/1 -> Product/1
  Gain4/1 -> Product2/2

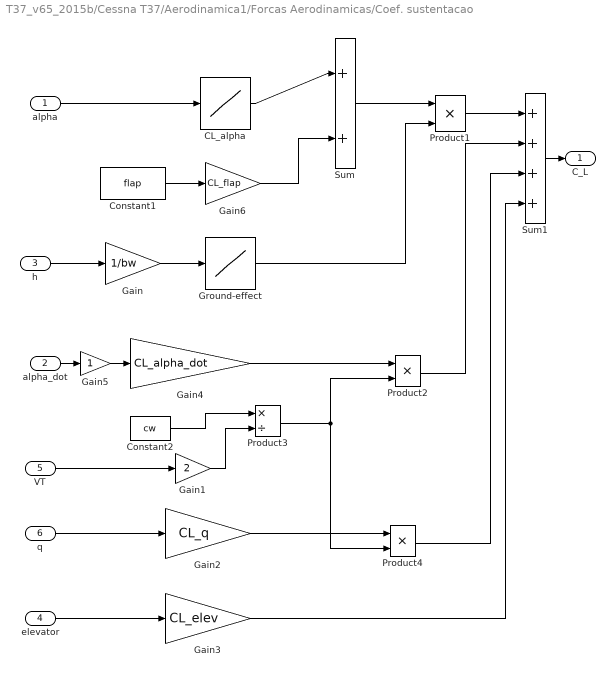
== system T37_v65_2015b/Cessna T37/Aerodinamica1/Forcas Aerodinamicas/Coef. sustentacao ==
  alpha : Inport
  alpha_dot : Inport  Port=2
  h : Inport  Port=3
  elevator : Inport  Port=4
  VT : Inport  Port=5
  q : Inport  Port=6
  CL_alpha : Lookup  InputValues=CL_alpha(:,1);  Table=CL_alpha(:,2);  LookUpMeth=Interpolation-Use End Values  SaturateOnIntegerOverflow=on
  Constant1 : Constant  Value=flap
  Constant2 : Constant  Value=cw
  Gain : Gain  Gain=1/bw  SaturateOnIntegerOverflow=on  OutDataTypeStr=Inherit: Same as input  ParamDataTypeStr=Inherit: Same as input
  Gain1 : Gain  Gain=2  SaturateOnIntegerOverflow=on  OutDataTypeStr=Inherit: Same as input  ParamDataTypeStr=Inherit: Same as input
  Gain2 : Gain  Gain=CL_q  SaturateOnIntegerOverflow=on  OutDataTypeStr=Inherit: Same as input  ParamDataTypeStr=Inherit: Same as input
  Gain3 : Gain  Gain=CL_elev  SaturateOnIntegerOverflow=on  OutDataTypeStr=Inherit: Same as input  ParamDataTypeStr=Inherit: Same as input
  Gain4 : Gain  Gain=CL_alpha_dot  SaturateOnIntegerOverflow=on  OutDataTypeStr=Inherit: Same as input  ParamDataTypeStr=Inherit: Same as input
  Gain5 : Gain  SaturateOnIntegerOverflow=on  OutDataTypeStr=Inherit: Same as input  ParamDataTypeStr=Inherit: Same as input
  Gain6 : Gain  Gain=CL_flap  SaturateOnIntegerOverflow=on  OutDataTypeStr=Inherit: Same as input  ParamDataTypeStr=Inherit: Same as input
  Ground-effect : Lookup  InputValues=CL_ground_effect(:,1);  Table=CL_ground_effect(:,2);  LookUpMeth=Interpolation-Use End Values  SaturateOnIntegerOverflow=on
  Product1 : Product  SaturateOnIntegerOverflow=on  OutDataTypeStr=Inherit: Same as first input
  Product2 : Product  SaturateOnIntegerOverflow=on  OutDataTypeStr=Inherit: Same as first input
  Product3 : Product  Inputs=*/  SaturateOnIntegerOverflow=on  OutDataTypeStr=Inherit: Same as first input
  Product4 : Product  SaturateOnIntegerOverflow=on  OutDataTypeStr=Inherit: Same as first input
  Sum : Sum  Inputs=|++  SaturateOnIntegerOverflow=on
  Sum1 : Sum  Inputs=++++  SaturateOnIntegerOverflow=on
  C_L : Outport
  wires:
  alpha/1 -> CL_alpha/1
  Sum/1 -> Product1/1
  Ground-effect/1 -> Product1/2
  Gain/1 -> Ground-effect/1
  h/1 -> Gain/1
  Product1/1 -> Sum1/1
  Sum1/1 -> C_L/1
  Gain4/1 -> Product2/1
  VT/1 -> Gain1/1
  Gain1/1 -> Product3/2
  alpha_dot/1 -> Gain5/1
  Constant2/1 -> Product3/1
  Product2/1 -> Sum1/2
  Product3/1 -> Product2/2, Product4/2
  Gain2/1 -> Product4/1
  Product4/1 -> Sum1/3
  q/1 -> Gain2/1
  elevator/1 -> Gain3/1
  Gain3/1 -> Sum1/4
  Gain5/1 -> Gain4/1
  Constant1/1 -> Gain6/1
  CL_alpha/1 -> Sum/1
  Gain6/1 -> Sum/2

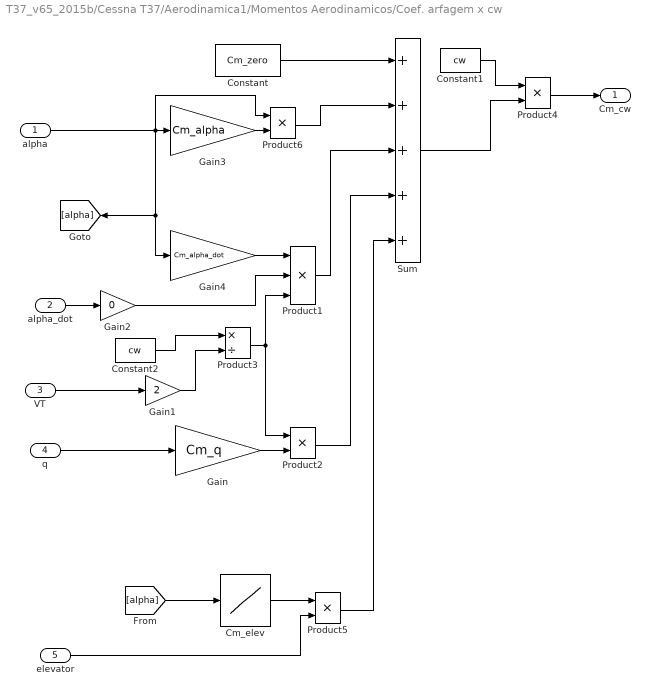
== system T37_v65_2015b/Cessna T37/Aerodinamica1/Momentos Aerodinamicos/Coef. arfagem x cw ==
  alpha : Inport
  alpha_dot : Inport  Port=2
  VT : Inport  Port=3
  q : Inport  Port=4
  elevator : Inport  Port=5
  Cm_elev : Lookup  InputValues=Cm_elev(:,1);  Table=Cm_elev(:,2);  SaturateOnIntegerOverflow=on
  Constant : Constant  Value=Cm_zero
  Constant1 : Constant  Value=cw
  Constant2 : Constant  Value=cw
  Gain : Gain  Gain=Cm_q  SaturateOnIntegerOverflow=on  OutDataTypeStr=Inherit: Same as input  ParamDataTypeStr=Inherit: Same as input
  Gain1 : Gain  Gain=2  SaturateOnIntegerOverflow=on  OutDataTypeStr=Inherit: Same as input  ParamDataTypeStr=Inherit: Same as input
  Gain2 : Gain  Gain=0  SaturateOnIntegerOverflow=on  OutDataTypeStr=Inherit: Same as input  ParamDataTypeStr=Inherit: Same as input
  Gain3 : Gain  Gain=Cm_alpha  SaturateOnIntegerOverflow=on  OutDataTypeStr=Inherit: Same as input  ParamDataTypeStr=Inherit: Same as input
  Gain4 : Gain  Gain=Cm_alpha_dot  SaturateOnIntegerOverflow=on  OutDataTypeStr=Inherit: Same as input  ParamDataTypeStr=Inherit: Same as input
  Product1 : Product  Inputs=***  SaturateOnIntegerOverflow=on  OutDataTypeStr=Inherit: Same as first input
  Product{2,4..6} (4 alike) : Product  Inputs=**  SaturateOnIntegerOverflow=on  OutDataTypeStr=Inherit: Same as first input
  Product3 : Product  Inputs=*/  SaturateOnIntegerOverflow=on  OutDataTypeStr=Inherit: Same as first input
  Sum : Sum  Inputs=+++++  SaturateOnIntegerOverflow=on
  Cm_cw : Outport
  wires:
  alpha/1 -> Gain3/1, Gain4/1, [alpha], Product6/1
  Constant1/1 -> Product4/1
  Sum/1 -> Product4/2
  Product4/1 -> Cm_cw/1
  Constant/1 -> Sum/1
  VT/1 -> Gain1/1
  Gain1/1 -> Product3/2
  Constant2/1 -> Product3/1
  Product1/1 -> Sum/3
  alpha_dot/1 -> Gain2/1
  Product3/1 -> Product1/3, Product2/1
  q/1 -> Gain/1
  Gain/1 -> Product2/2
  Product2/1 -> Sum/4
  [alpha] -> Cm_elev/1
  Cm_elev/1 -> Product5/1
  elevator/1 -> Product5/2
  Gain2/1 -> Product1/2
  Product6/1 -> Sum/2
  Gain3/1 -> Product6/2
  Gain4/1 -> Product1/1
  Product5/1 -> Sum/5

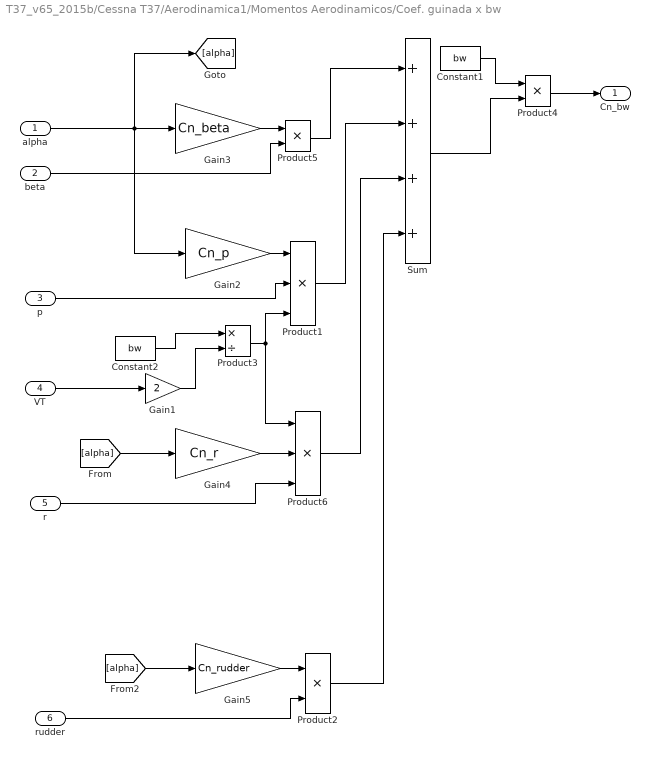
== system T37_v65_2015b/Cessna T37/Aerodinamica1/Momentos Aerodinamicos/Coef. guinada x bw ==
  alpha : Inport
  beta : Inport  Port=2
  p : Inport  Port=3
  VT : Inport  Port=4
  r : Inport  Port=5
  rudder : Inport  Port=6
  Constant1 : Constant  Value=bw
  Constant2 : Constant  Value=bw
  Gain1 : Gain  Gain=2  SaturateOnIntegerOverflow=on  OutDataTypeStr=Inherit: Same as input  ParamDataTypeStr=Inherit: Same as input
  Gain2 : Gain  Gain=Cn_p  SaturateOnIntegerOverflow=on  OutDataTypeStr=Inherit: Same as input  ParamDataTypeStr=Inherit: Same as input
  Gain3 : Gain  Gain=Cn_beta  SaturateOnIntegerOverflow=on  OutDataTypeStr=Inherit: Same as input  ParamDataTypeStr=Inherit: Same as input
  Gain4 : Gain  Gain=Cn_r  SaturateOnIntegerOverflow=on  OutDataTypeStr=Inherit: Same as input  ParamDataTypeStr=Inherit: Same as input
  Gain5 : Gain  Gain=Cn_rudder  SaturateOnIntegerOverflow=on  OutDataTypeStr=Inherit: Same as input  ParamDataTypeStr=Inherit: Same as input
  Product1 : Product  Inputs=***  SaturateOnIntegerOverflow=on  OutDataTypeStr=Inherit: Same as first input
  Product2 : Product  Inputs=**  SaturateOnIntegerOverflow=on  OutDataTypeStr=Inherit: Same as first input
  Product3 : Product  Inputs=*/  SaturateOnIntegerOverflow=on  OutDataTypeStr=Inherit: Same as first input
  Product4 : Product  Inputs=**  SaturateOnIntegerOverflow=on  OutDataTypeStr=Inherit: Same as first input
  Product5 : Product  Inputs=**  SaturateOnIntegerOverflow=on  OutDataTypeStr=Inherit: Same as first input
  Product6 : Product  Inputs=***  SaturateOnIntegerOverflow=on  OutDataTypeStr=Inherit: Same as first input
  Sum : Sum  Inputs=++++  SaturateOnIntegerOverflow=on
  Cn_bw : Outport
  wires:
  alpha/1 -> Gain2/1, Gain3/1, [alpha]
  Constant1/1 -> Product4/1
  Sum/1 -> Product4/2
  Product4/1 -> Cn_bw/1
  VT/1 -> Gain1/1
  Gain1/1 -> Product3/2
  Constant2/1 -> Product3/1
  beta/1 -> Product5/2
  Product5/1 -> Sum/1
  Product3/1 -> Product1/3, Product6/1
  p/1 -> Product1/2
  Product1/1 -> Sum/2
  r/1 -> Product6/3
  Product6/1 -> Sum/3
  rudder/1 -> Product2/2
  Gain3/1 -> Product5/1
  Gain2/1 -> Product1/1
  Gain4/1 -> Product6/2
  [alpha] -> Gain4/1
  Gain5/1 -> Product2/1
  [alpha] -> Gain5/1
  Product2/1 -> Sum/4

== system T37_v65_2015b/Cessna T37/Aerodinamica1/Momentos Aerodinamicos/Coef. rolamento x bw ==
  alpha : Inport
  beta : Inport  Port=2
  VT : Inport  Port=3
  p : Inport  Port=4
  r : Inport  Port=5
  aileron : Inport  Port=6
  rudder : Inport  Port=7
  Cm_elev : Lookup  InputValues=Cl_ail(:,1);  Table=Cl_ail(:,2);  SaturateOnIntegerOverflow=on
  Constant1 : Constant  Value=bw
  Constant2 : Constant  Value=bw
  Gain1 : Gain  Gain=2  SaturateOnIntegerOverflow=on  OutDataTypeStr=Inherit: Same as input  ParamDataTypeStr=Inherit: Same as input
  Gain2 : Gain  Gain=Cl_rudder  SaturateOnIntegerOverflow=on  OutDataTypeStr=Inherit: Same as input  ParamDataTypeStr=Inherit: Same as input
  Gain3 : Gain  Gain=Cl_beta  SaturateOnIntegerOverflow=on  OutDataTypeStr=Inherit: Same as input  ParamDataTypeStr=Inherit: Same as input
  Gain4 : Gain  Gain=Cl_p  SaturateOnIntegerOverflow=on  OutDataTypeStr=Inherit: Same as input  ParamDataTypeStr=Inherit: Same as input
  Gain5 : Gain  Gain=Cl_r  SaturateOnIntegerOverflow=on  OutDataTypeStr=Inherit: Same as input  ParamDataTypeStr=Inherit: Same as input
  Product1 : Product  Inputs=3  SaturateOnIntegerOverflow=on  OutDataTypeStr=Inherit: Same as first input
  Product2 : Product  Inputs=3  SaturateOnIntegerOverflow=on  OutDataTypeStr=Inherit: Same as first input
  Product3 : Product  Inputs=*/  SaturateOnIntegerOverflow=on  OutDataTypeStr=Inherit: Same as first input
  Product4 : Product  Inputs=**  SaturateOnIntegerOverflow=on  OutDataTypeStr=Inherit: Same as first input
  Product5 : Product  SaturateOnIntegerOverflow=on  OutDataTypeStr=Inherit: Same as first input
  Sum : Sum  Inputs=+++++  SaturateOnIntegerOverflow=on
  Cl_bw : Outport
  wires:
  VT/1 -> Gain1/1
  Gain1/1 -> Product3/2
  Constant2/1 -> Product3/1
  Product3/1 -> Product1/1, Product2/1
  Gain4/1 -> Product1/2
  p/1 -> Product1/3
  r/1 -> Product2/3
  aileron/1 -> Cm_elev/1
  rudder/1 -> Gain2/1
  Product1/1 -> Sum/2
  Product2/1 -> Sum/3
  Cm_elev/1 -> Sum/4
  Gain2/1 -> Sum/5
  Constant1/1 -> Product4/1
  Sum/1 -> Product4/2
  Product4/1 -> Cl_bw/1
  beta/1 -> Product5/1
  alpha/1 -> Gain5/1, Gain4/1, Gain3/1
  Product5/1 -> Sum/1
  Gain3/1 -> Product5/2
  Gain5/1 -> Product2/2
